simulink model "TP3_2_3"  (R2018a)
settings: Solver=ode45  StartTime=0.0  StopTime=1  RelTol=1e-3
libraries: dsparch4 x6, dspsrcs4 x1
settings Model: Creator=10RS6N  LastModifiedBy=10RS5
settings SolverCC: AutoInsertRateTranBlk=on
settings DataIOCC: SaveFormat=StructureWithTime  ReturnWorkspaceOutputs=on
settings OptimizationCC: LifeSpan=inf
settings DebuggingCC: SFExecutionAtInitializationDiag=none
settings HardwareCC: ProdBitPerSizeT=32  ProdBitPerPtrDiffT=32  ProdWordSize=32  ProdHWDeviceType=Specified
settings SFSimCC: SimUseLocalCustomCode=on
settings RTWCC: RTWUseLocalCustomCode=on
settings CodeAppCC: StateflowObjectComments=on

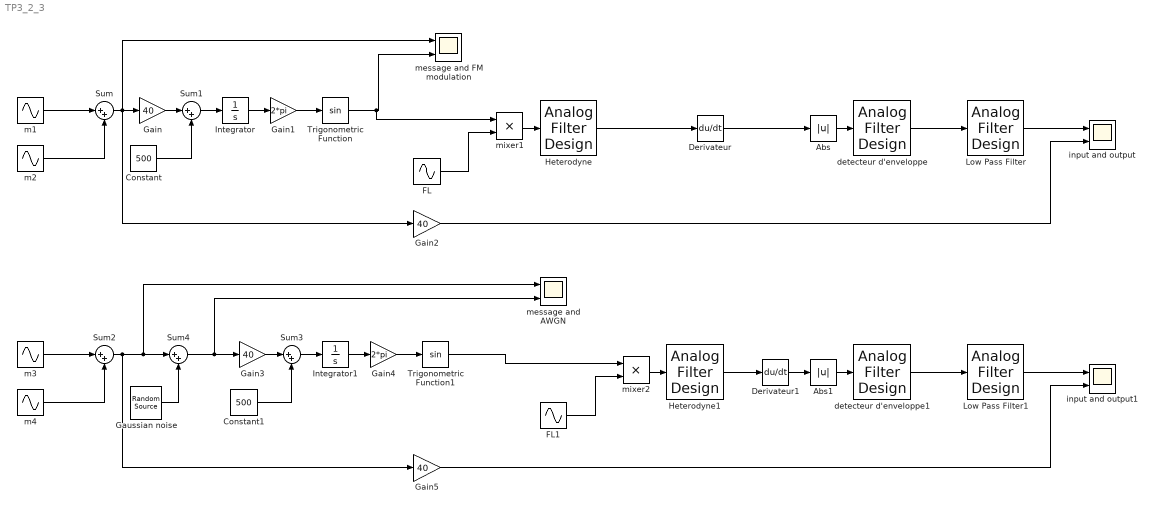
== system TP3_2_3 ==
  Abs : Abs
  Abs1 : Abs
  Constant : Constant  Value=500
  Constant1 : Constant  Value=500
  Derivateur : Derivative
  Derivateur1 : Derivative
  FL : Sin  Frequency=300*2*pi  SampleTime=0
  FL1 : Sin  Frequency=300*2*pi  SampleTime=0
  Gain{,2..3,5} (4 alike) : Gain  Gain=40
  Gain1 : Gain  Gain=2*pi
  Gain4 : Gain  Gain=2*pi
  Gaussian noise : dspsrcs4/Random Source  SrcType=Gaussian  NormMethod=Ziggurat  CltLength=12  MinVal=0  MaxVal=1  MeanVal=0  VarVal=1  RepMode=Not repeatable  rawSeed=1  IsInherit=off  SampMode=Continuous  SampTime=1  SampFrame=1  DataType=Double  OutComplex=Real  OutputFrames=off
  Heterodyne : dsparch4/Analog Filter Design  method=Butterworth  filttype=Bandpass  N=8  Wlo=100*2*pi  Whi=500*2*pi  Rp=2  Rs=40
  Heterodyne1 : dsparch4/Analog Filter Design  method=Butterworth  filttype=Bandpass  N=8  Wlo=100*2*pi  Whi=500*2*pi  Rp=2  Rs=40
  Integrator : Integrator
  Integrator1 : Integrator
  Low Pass Filter : dsparch4/Analog Filter Design  method=Butterworth  filttype=Lowpass  N=10  Wlo=13*2*pi  Whi=1885  Rp=2  Rs=40
  Low Pass Filter1 : dsparch4/Analog Filter Design  method=Butterworth  filttype=Lowpass  N=10  Wlo=13*2*pi  Whi=1885  Rp=2  Rs=40
  Sum{,1..4} (5 alike) : Sum  Inputs=|++
  Trigonometric Function : Trigonometry
  Trigonometric Function1 : Trigonometry
  detecteur d'enveloppe : dsparch4/Analog Filter Design  method=Butterworth  filttype=Lowpass  N=6  Wlo=100*2*pi  Whi=1885  Rp=2  Rs=40
  detecteur d'enveloppe1 : dsparch4/Analog Filter Design  method=Butterworth  filttype=Lowpass  N=6  Wlo=100*2*pi  Whi=1885  Rp=2  Rs=40
  input and output : Scope  NumInputPorts=2
  input and output1 : Scope  NumInputPorts=2
  m1 : Sin  Frequency=31.41  SampleTime=0
  m2 : Sin  Amplitude=0.5  Frequency=62.83  SampleTime=0
  m3 : Sin  Frequency=31.41  SampleTime=0
  m4 : Sin  Amplitude=0.5  Frequency=62.83  SampleTime=0
  message and AWGN : Scope  NumInputPorts=2
  message and FM modulation : Scope  NumInputPorts=2
  mixer1 : Product
  mixer2 : Product
  wires:
  m2/1 -> Sum/2
  m1/1 -> Sum/1
  Gain/1 -> Sum1/1
  Constant/1 -> Sum1/2
  Sum1/1 -> Integrator/1
  Gain1/1 -> Trigonometric Function/1
  Trigonometric Function/1 -> message and FM modulation/2, mixer1/1
  mixer1/1 -> Heterodyne/1
  FL/1 -> mixer1/2
  Abs/1 -> detecteur d'enveloppe/1
  detecteur d'enveloppe/1 -> Low Pass Filter/1
  Low Pass Filter/1 -> input and output/1
  Heterodyne/1 -> Derivateur/1
  Derivateur/1 -> Abs/1
  Integrator/1 -> Gain1/1
  Sum/1 -> Gain2/1, message and FM modulation/1, Gain/1
  Gain2/1 -> input and output/2
  Gain5/1 -> input and output1/2
  Sum2/1 -> message and AWGN/1, Sum4/1, Gain5/1
  Integrator1/1 -> Gain4/1
  Derivateur1/1 -> Abs1/1
  Heterodyne1/1 -> Derivateur1/1
  Low Pass Filter1/1 -> input and output1/1
  detecteur d'enveloppe1/1 -> Low Pass Filter1/1
  Abs1/1 -> detecteur d'enveloppe1/1
  FL1/1 -> mixer2/2
  mixer2/1 -> Heterodyne1/1
  Gain4/1 -> Trigonometric Function1/1
  Sum3/1 -> Integrator1/1
  Constant1/1 -> Sum3/2
  Gain3/1 -> Sum3/1
  m3/1 -> Sum2/1
  m4/1 -> Sum2/2
  Trigonometric Function1/1 -> mixer2/1
  Sum4/1 -> message and AWGN/2, Gain3/1
  Gaussian noise/1 -> Sum4/2
